simulink model "LTI_vs_LPV_vs_NL_realimentado_NL"  (R2020a)
settings: Solver=VariableStepAuto  StartTime=0.0  StopTime=10.0  RelTol=1e-3
values from neighbouring files (symbols this model uses):
  A = [ 0        1               0 ... (first row only)    [AnalisisDeEstabilidad.m]    (also in Consigna_de_pos.m = [t_1^3,t_1^2,t_1,1; Controlabilidad.m = [0 ,       1      ,         0; Funciones_de_Transferencia.m = [ 0         1                           0; LTI_vs_LPV_vs_NL_realimentado.m = [0                                                       1  )
  alpha_cu = 3.9e-3    (= 0.0039)    [AnalisisDeEstabilidad.m]    (also in LTI_vs_LPV_vs_NL_realimentado.m; Modelo_linealizado.m)
  B = [0              0 ... (first row only)    [AnalisisDeEstabilidad.m]    (also in Consigna_de_pos.m = [theta_m1; theta_m2; 0 ;0]; Controlabilidad.m = [0;0;1/Lq]; LTI_vs_LPV_vs_NL_realimentado.m = [0      0       0           0           0; Modelo_linealizado.m = [0,0,0,0,0)
  b_eq = b_m + b_l/(r^2)    (= 2.19444444444e-05)    [LTI_vs_LPV_vs_NL_realimentado.m]    (also in Modelo_linealizado.m)
  C_ts = 0.818    [LTI_vs_LPV_vs_NL_realimentado.m]    (also in Modelo_linealizado.m)
  i_0s_o = double(solutions.i_0so(1))    [LTI_vs_LPV_vs_NL_realimentado.m]
  i_ds_o = double(solutions.i_tot(1)*cos(beta))    [LTI_vs_LPV_vs_NL_realimentado.m]    (also in Modelo_linealizado.m = 0)
  i_qs_o = double(solutions.i_tot(1)*sin(beta))    [LTI_vs_LPV_vs_NL_realimentado.m]    (also in Modelo_linealizado.m = 0)
  J_eq = J_m + J_l/(r^2)    (= 1.97847222222e-05)    [LTI_vs_LPV_vs_NL_realimentado.m]    (also in Modelo_linealizado.m)
  L_d = 6.6/1000    (= 0.0066)    [Curvas_carc.m]    (also in LTI_vs_LPV_vs_NL_realimentado.m; Modelo_linealizado.m)
  L_ls = 0.8/1000    (= 0.0008)    [LTI_vs_LPV_vs_NL_realimentado.m]    (also in Modelo_linealizado.m)
  L_q = 5.8/1000    (= 0.0058)    [Curvas_carc.m]    (also in LTI_vs_LPV_vs_NL_realimentado.m; Modelo_linealizado.m)
  lambda_m = 0.01546    [Curvas_carc.m]    (also in LTI_vs_LPV_vs_NL_realimentado.m = 0.016; Modelo_linealizado.m = 0.016)
  omega_m_o = double(solutions.omega_mo(1))    [LTI_vs_LPV_vs_NL_realimentado.m]    (also in Modelo_linealizado.m = 0)
  P_p = 3    [Curvas_carc.m]    (also in LTI_vs_LPV_vs_NL_realimentado.m)
  Pp = 3    [AnalisisDeEstabilidad.m]    (also in LTI_vs_LPV_vs_NL_realimentado.m; Modelo_linealizado.m; parametros.m)
  r = 120    [AnalisisDeEstabilidad.m]    (also in LTI_vs_LPV_vs_NL_realimentado.m; Modelo_linealizado.m; parametros.m)
  R_s = 1.02    [Curvas_carc.m]    (also in LTI_vs_LPV_vs_NL_realimentado.m = R_s_o; Modelo_linealizado.m = 0.348)
  R_sREF = R_sref    (= 1.02)    [LTI_vs_LPV_vs_NL_realimentado.m]
  R_ts_amb = 146.7    [LTI_vs_LPV_vs_NL_realimentado.m]    (also in Modelo_linealizado.m)
  T_amb = T_amb_o    (= 25)    [LTI_vs_LPV_vs_NL_realimentado.m]
  T_amb_o = 25    [LTI_vs_LPV_vs_NL_realimentado.m]    (also in Modelo_linealizado.m = -15:10:40)
  T_l_o = 0    [LTI_vs_LPV_vs_NL_realimentado.m]
  T_s_o = double(solutions.T_so(1))    [LTI_vs_LPV_vs_NL_realimentado.m]    (also in Modelo_linealizado.m = 40)
  T_sREF = T_sref    (= 40)    [LTI_vs_LPV_vs_NL_realimentado.m]
  theta_m_o = r*pi/12    (= 31.4159265359)    [LTI_vs_LPV_vs_NL_realimentado.m]    (also in Modelo_linealizado.m = 0)
  v_0s = v_0s_o    (= 0)    [LTI_vs_LPV_vs_NL_realimentado.m]    (also in Modelo_linealizado.m)
  v_0s_o = 0    [LTI_vs_LPV_vs_NL_realimentado.m]
  v_ds = 10    [Curvas_carc.m]    (also in LTI_vs_LPV_vs_NL_realimentado.m = 0)
  v_ds_o = double(solutions.v_dso(1))    [LTI_vs_LPV_vs_NL_realimentado.m]
  v_qs_o = double(solutions.v_qso(1))    [LTI_vs_LPV_vs_NL_realimentado.m]
undefined symbols (not defined in the file or in its folder): sigbuilder_block
settings Model: Creator=Juan  LastModifiedBy=Juan

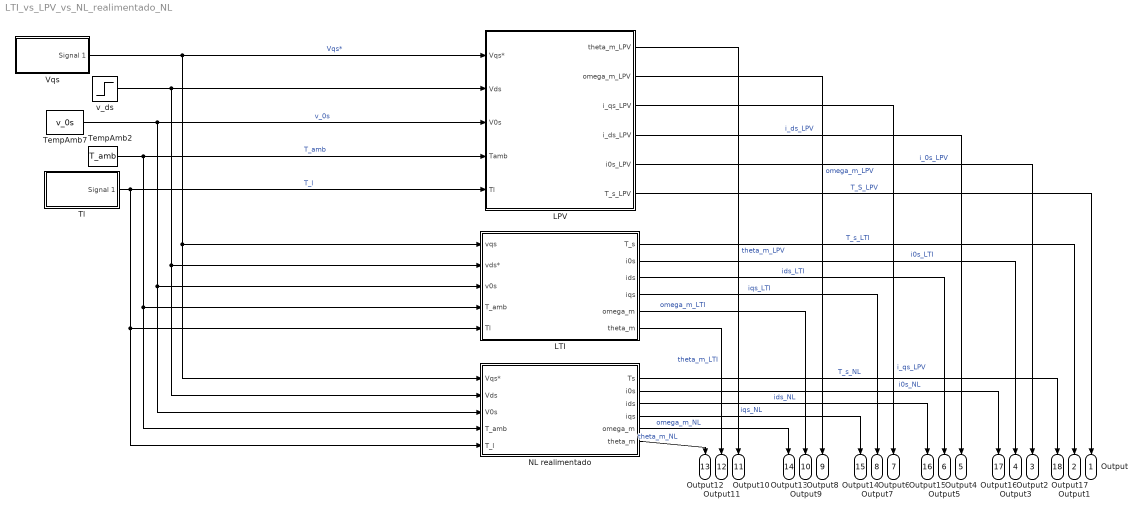
== system LTI_vs_LPV_vs_NL_realimentado_NL ==
  LPV : Subsystem
  LTI : Subsystem
  NL realimentado : Subsystem
  TempAmb2 : Constant  Value=T_amb
  TempAmb7 : Constant  Value=v_0s
  Tl : Subsystem  Tag=STV Subsys  LoadFcn=sigbuilder_block('load');  StartFcn=sigbuilder_block('start');  StopFcn=sigbuilder_block('stop');  ClipboardFcn=sigbuilder_block('clipboard');  mask(Sigbuilder block){tuvar=[0:10]}
      mask help: Simulink:masks:SigbuilderBlock_MD
      mask init:
      | if ~strcmp(get_param(bdroot(gcbh),'SimulationStatus'),'stopped') tuvar = sigbuilder_block('maskInit'); end
      settings: CopyFcn=sigbuilder_block('copy');  DeleteFcn=sigbuilder_block('delete');  ModelCloseFcn=sigbuilder_block('modelClose');  PreSaveFcn=sigbuilder_block('preSave');  PauseFcn=sigbuilder_block('pause');  ContinueFcn=sigbuilder_block('continue');  NameChangeFcn=sigbuilder_block('namechange');  OpenFcn=sigbuilder_block('open',[0 36 1152 555.6 ]);  CloseFcn=sigbuilder_block('close');
      mask Display: plot(0, 0, 100, 100,[2, 2, 32, 32, 2], [68, 8, 8, 68, 68],[32, 2], [38, 38], [32, 19, 2],[53, 60, 44], [32, 17, 17, 2],[16, 16, 31, 31]);txt = getActiveGroup(gcbh);text(2, 100, txt,'verticalAlignment', 'top');
  Vqs : Subsystem  Tag=STV Subsys  LoadFcn=sigbuilder_block('load');  StartFcn=sigbuilder_block('start');  StopFcn=sigbuilder_block('stop');  ClipboardFcn=sigbuilder_block('clipboard');  mask(Sigbuilder block){tuvar=[0:10]}
      mask help: Simulink:masks:SigbuilderBlock_MD
      mask init:
      | if ~strcmp(get_param(bdroot(gcbh),'SimulationStatus'),'stopped') tuvar = sigbuilder_block('maskInit'); end
      settings: CopyFcn=sigbuilder_block('copy');  DeleteFcn=sigbuilder_block('delete');  ModelCloseFcn=sigbuilder_block('modelClose');  PreSaveFcn=sigbuilder_block('preSave');  PauseFcn=sigbuilder_block('pause');  ContinueFcn=sigbuilder_block('continue');  NameChangeFcn=sigbuilder_block('namechange');  OpenFcn=sigbuilder_block('open',[5.4 36 1141.2 516.6 ]);  CloseFcn=sigbuilder_block('close');
      mask Display: plot(0, 0, 100, 100,[2, 2, 32, 32, 2], [68, 8, 8, 68, 68],[32, 2], [38, 38], [32, 19, 2],[53, 60, 44], [32, 17, 17, 2],[16, 16, 31, 31]);txt = getActiveGroup(gcbh);text(2, 100, txt,'verticalAlignment', 'top');
  v_ds : Step  After=v_ds  SampleTime=0
  Output : Outport
  Output1 : Outport  Port=2
  Output2 : Outport  Port=3
  Output3 : Outport  Port=4
  Output4 : Outport  Port=5
  Output5 : Outport  Port=6
  Output6 : Outport  Port=7
  Output7 : Outport  Port=8
  Output8 : Outport  Port=9
  Output9 : Outport  Port=10
  Output10 : Outport  Port=11
  Output11 : Outport  Port=12
  Output12 : Outport  Port=13
  Output13 : Outport  Port=14
  Output14 : Outport  Port=15
  Output15 : Outport  Port=16
  Output16 : Outport  Port=17
  Output17 : Outport  Port=18
  wires:
  LTI/3(ids) -> Output5/1  "ids_LTI"
  LTI/5(omega_m) -> Output9/1  "omega_m_LTI"
  LTI/1(T_s) -> Output1/1  "T_s_LTI"
  LTI/4(iqs) -> Output7/1  "iqs_LTI"
  LTI/2(i0s) -> Output3/1  "i0s_LTI"
  TempAmb7/1 -> NL realimentado/3(V0s), LTI/3(v0s), LPV/3(V0s)  "v_0s"
  TempAmb2/1 -> NL realimentado/4(T_amb), LTI/4(T_amb), LPV/4(Tamb)  "T_amb"
  LTI/6(theta_m) -> Output11/1  "theta_m_LTI"
  v_ds/1 -> NL realimentado/2(Vds), LTI/2(vds*), LPV/2(Vds)
  Tl/1(Signal 1) -> LPV/5(Tl), NL realimentado/5(T_l), LTI/5(Tl)  "T_l"
  Vqs/1(Signal 1) -> NL realimentado/1(Vqs*), LTI/1(vqs), LPV/1(Vqs*)  "Vqs*"
  LPV/1(theta_m_LPV) -> Output10/1  "theta_m_LPV"
  LPV/2(omega_m_LPV) -> Output8/1  "omega_m_LPV"
  LPV/3(i_qs_LPV) -> Output6/1  "i_qs_LPV"
  LPV/4(i_ds_LPV) -> Output4/1  "i_ds_LPV"
  LPV/5(i0s_LPV) -> Output2/1  "i_0s_LPV"
  LPV/6(T_s_LPV) -> Output/1  "T_S_LPV"
  NL realimentado/6(theta_m) -> Output12/1  "theta_m_NL"
  NL realimentado/5(omega_m) -> Output13/1  "omega_m_NL"
  NL realimentado/4(iqs) -> Output14/1  "iqs_NL"
  NL realimentado/3(ids) -> Output15/1  "ids_NL"
  NL realimentado/2(i0s) -> Output16/1  "i0s_NL"
  NL realimentado/1(Ts) -> Output17/1  "T_s_NL"

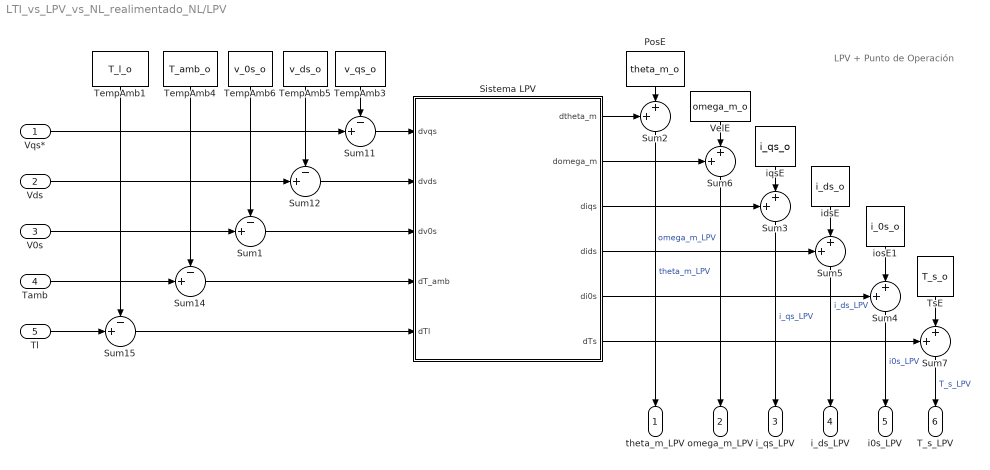
== system LTI_vs_LPV_vs_NL_realimentado_NL/LPV ==
  note: LPV + Punto de Operación
  Vqs* : Inport
  Vds : Inport  Port=2
  V0s : Inport  Port=3
  Tamb : Inport  Port=4
  Tl : Inport  Port=5
  PosE : Constant  Value=theta_m_o
  Sistema LPV : Subsystem
  Sum{1,11..12,14..15} (5 alike) : Sum  Inputs=-+|
  Sum{2..7} (6 alike) : Sum  Inputs=++|
  TempAmb1 : Constant  Value=T_l_o
  TempAmb3 : Constant  Value=v_qs_o
  TempAmb4 : Constant  Value=T_amb_o
  TempAmb5 : Constant  Value=v_ds_o
  TempAmb6 : Constant  Value=v_0s_o
  TsE : Constant  Value=T_s_o
  VelE : Constant  Value=omega_m_o
  idsE : Constant  Value=i_ds_o
  iosE1 : Constant  Value=i_0s_o
  iqsE : Constant  Value=i_qs_o
  theta_m_LPV : Outport
  omega_m_LPV : Outport  Port=2
  i_qs_LPV : Outport  Port=3
  i_ds_LPV : Outport  Port=4
  i0s_LPV : Outport  Port=5
  T_s_LPV : Outport  Port=6
  wires:
  V0s/1 -> Sum1/2
  Sum12/1 -> Sistema LPV/2(dvds)
  Sum1/1 -> Sistema LPV/3(dv0s)
  Sum5/1 -> i_ds_LPV/1  "i_ds_LPV"
  iosE1/1 -> Sum4/2
  TempAmb4/1 -> Sum14/1
  Sistema LPV/4(dids) -> Sum5/1
  TempAmb6/1 -> Sum1/1
  Tamb/1 -> Sum14/2
  iqsE/1 -> Sum3/2
  TsE/1 -> Sum7/2
  TempAmb5/1 -> Sum12/1
  idsE/1 -> Sum5/2
  TempAmb1/1 -> Sum15/1
  Sum14/1 -> Sistema LPV/4(dT_amb)
  Sistema LPV/6(dTs) -> Sum7/1
  Sum11/1 -> Sistema LPV/1(dvqs)
  Sistema LPV/2(domega_m) -> Sum6/1
  Sum15/1 -> Sistema LPV/5(dTl)
  Sistema LPV/5(di0s) -> Sum4/1
  Vds/1 -> Sum12/2
  VelE/1 -> Sum6/2
  Sum6/1 -> omega_m_LPV/1  "omega_m_LPV"
  PosE/1 -> Sum2/2
  Sistema LPV/1(dtheta_m) -> Sum2/1
  Sistema LPV/3(diqs) -> Sum3/1
  TempAmb3/1 -> Sum11/1
  Tl/1 -> Sum15/2
  Sum4/1 -> i0s_LPV/1  "i0s_LPV"
  Sum3/1 -> i_qs_LPV/1  "i_qs_LPV"
  Sum2/1 -> theta_m_LPV/1  "theta_m_LPV"
  Sum7/1 -> T_s_LPV/1  "T_s_LPV"
  Vqs*/1 -> Sum11/2

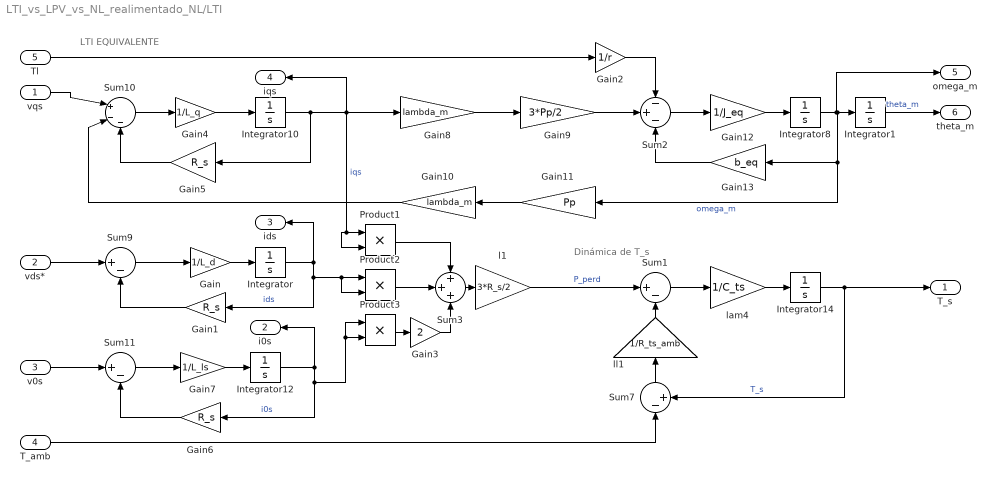
== system LTI_vs_LPV_vs_NL_realimentado_NL/LTI ==
  note: Dinámica de T_s
  note: LTI EQUIVALENTE
  vqs : Inport
  vds* : Inport  Port=2
  v0s : Inport  Port=3
  T_amb : Inport  Port=4
  Tl : Inport  Port=5
  Gain : Gain  Gain=1/L_d
  Gain1 : Gain  Gain=R_s
  Gain10 : Gain  Gain=lambda_m
  Gain11 : Gain  Gain=Pp
  Gain12 : Gain  Gain=1/J_eq
  Gain13 : Gain  Gain=b_eq
  Gain2 : Gain  Gain=1/r
  Gain3 : Gain  Gain=2
  Gain4 : Gain  Gain=1/L_q
  Gain5 : Gain  Gain=R_s
  Gain6 : Gain  Gain=R_s
  Gain7 : Gain  Gain=1/L_ls
  Gain8 : Gain  Gain=lambda_m
  Gain9 : Gain  Gain=3*Pp/2
  Integrator{,1,8,10,12} (5 alike) : Integrator
  Integrator14 : Integrator  InitialCondition=T_amb
  Product1 : Product
  Product2 : Product
  Product3 : Product
  Sum1 : Sum  Inputs=|+-
  Sum10 : Sum  Inputs=|+--
  Sum11 : Sum  Inputs=|+-
  Sum2 : Sum  Inputs=-+-
  Sum3 : Sum  Inputs=+++
  Sum7 : Sum  Inputs=|-+
  Sum9 : Sum  Inputs=|+-
  l1 : Gain  Gain=3*R_s/2
  lam4 : Gain  Gain=1/C_ts
  ll1 : Gain  Gain=1/R_ts_amb
  T_s : Outport
  i0s : Outport  Port=2
  ids : Outport  Port=3
  iqs : Outport  Port=4
  omega_m : Outport  Port=5
  theta_m : Outport  Port=6
  wires:
  Integrator/1 -> ids/1, Gain1/1, Product2/2, Product2/1  "ids"
  Sum7/1 -> ll1/1
  Gain5/1 -> Sum10/3
  Sum11/1 -> Gain7/1
  Gain7/1 -> Integrator12/1
  Product1/1 -> Sum3/1
  Gain13/1 -> Sum2/3
  Integrator8/1 -> omega_m/1, Integrator1/1, Gain11/1, Gain13/1  "omega_m"
  Gain6/1 -> Sum11/2
  Gain4/1 -> Integrator10/1
  Gain8/1 -> Gain9/1
  Gain/1 -> Integrator/1
  Integrator12/1 -> Product3/1, Product3/2, Gain6/1, i0s/1  "i0s"
  Integrator10/1 -> Product1/2, Product1/1, iqs/1, Gain8/1, Gain5/1  "iqs"
  Gain1/1 -> Sum9/2
  Tl/1 -> Gain2/1
  v0s/1 -> Sum11/1
  Gain11/1 -> Gain10/1
  lam4/1 -> Integrator14/1
  Gain10/1 -> Sum10/2
  T_amb/1 -> Sum7/1
  Gain2/1 -> Sum2/1
  Sum1/1 -> lam4/1
  Integrator14/1 -> Sum7/2, T_s/1  "T_s"
  l1/1 -> Sum1/1  "P_perd"
  vds*/1 -> Sum9/1
  Gain12/1 -> Integrator8/1
  Product2/1 -> Sum3/2
  Sum9/1 -> Gain/1
  Gain3/1 -> Sum3/3
  Gain9/1 -> Sum2/2
  Integrator1/1 -> theta_m/1  "theta_m"
  Product3/1 -> Gain3/1
  vqs/1 -> Sum10/1
  Sum2/1 -> Gain12/1
  Sum10/1 -> Gain4/1
  ll1/1 -> Sum1/2
  Sum3/1 -> l1/1

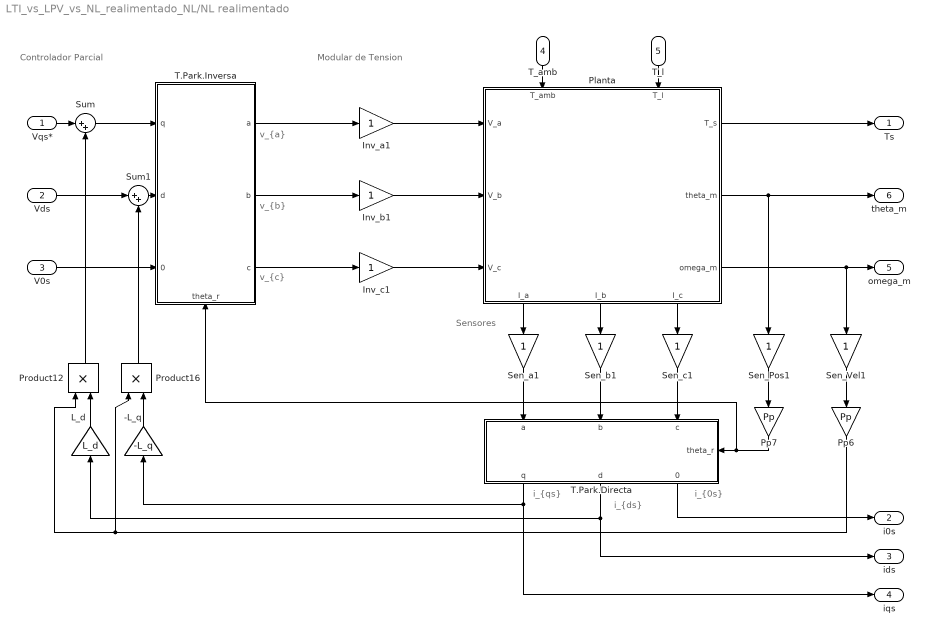
== system LTI_vs_LPV_vs_NL_realimentado_NL/NL realimentado ==
  note: i_{qs}
  note: i_{ds}
  note: Modular de Tension
  note: v_{c}
  note: Controlador Parcial
  note: Sensores
  note: v_{a}
  note: i_{0s}
  note: v_{b}
  Vqs* : Inport
  Vds : Inport  Port=2
  V0s : Inport  Port=3
  T_amb : Inport  Port=4
  T_l : Inport  Port=5
  -L_q : Gain  Gain=-L_q
  Inv_a1 : Gain
  Inv_b1 : Gain
  Inv_c1 : Gain
  L_d : Gain  Gain=L_d
  Planta : Subsystem
      settings: PortSchema="{\"entries\":[{\"content\":{\"sides\":[{\"content\":{\"connectorIds\":[\"In1\",\"In2\",\"In3\"]},\"type\":\"ConnectorPlacement.EquallySpacedRectSide\",\"uuid\":\"baf32630-7abf-43de-8d1d-ef19bce8ef09\"},{\"content\":{\"connectorIds\":[\"Out1\",\"Out2\",\"Out3\"],\"side\":\"RIGHT\"},\"type\":\"ConnectorPlacement.EquallySpacedRectSide\",\"uuid\":\"8343cc29-d6ed-46ed-8bbc-86cce19f52c3\"},{\"content\":{\"connectorIds\":[\"In4\",\"In5\"],\"side\":\"TOP\"},\"type\":\"ConnectorPlacement.EquallySpacedRectSide\",\"uuid\":\"0b8be76f-f25b-4801-8835-92ed2105f393\"},{\"content\":{\"connectorIds\":[\"Out4\",\"Out5\",\"Out6\"],\"side\":\"BOTTOM\"},\"type\":\"ConnectorPlacement.EquallySpacedRectSide\",\"uuid\":\"fe3e13b1-008f-430e-9d12-27931368b9b5\"}]},\"type\":\"ConnectorPlacement.EquallySpacedConnector\",\"uuid\":\"84d47617-2d56-43e0-a9a1-133a35a1552a\"}],\"packageUris\":[\"http://schema.mathworks.com/mf0/Connector/19700101\"],\"version\":\"1.0\"}"
  Pp6 : Gain  Gain=Pp
  Pp7 : Gain  Gain=Pp
  Product12 : Product
  Product16 : Product
  Sen_Pos1 : Gain
  Sen_Vel1 : Gain
  Sen_a1 : Gain
  Sen_b1 : Gain
  Sen_c1 : Gain
  Sum : Sum  Inputs=|++
  Sum1 : Sum  Inputs=|++
  T.Park.Directa : Subsystem
      settings: PortSchema="{\"entries\":[{\"content\":{\"sides\":[{\"content\":{\"connectorIds\":[\"In1\",\"In2\",\"In3\"]},\"type\":\"ConnectorPlacement.EquallySpacedRectSide\",\"uuid\":\"2bfbe7ef-652a-4797-b13c-b84c243bd68c\"},{\"content\":{\"connectorIds\":[\"Out1\",\"Out2\",\"Out3\"],\"side\":\"RIGHT\"},\"type\":\"ConnectorPlacement.EquallySpacedRectSide\",\"uuid\":\"075def0e-c436-44dc-ba25-82cf6ffae869\"},{\"content\":{\"connectorIds\":[],\"side\":\"TOP\"},\"type\":\"ConnectorPlacement.EquallySpacedRectSide\",\"uuid\":\"95d81334-e332-4f04-a2cb-c4692f91809c\"},{\"content\":{\"connectorIds\":[\"In4\"],\"side\":\"BOTTOM\"},\"type\":\"ConnectorPlacement.EquallySpacedRectSide\",\"uuid\":\"85b95360-e43d-49d1-a18f-690334b045e6\"}]},\"type\":\"ConnectorPlacement.EquallySpacedConnector\",\"uuid\":\"b90f9cad-0277-459c-bcac-17172872a787\"}],\"packageUris\":[\"http://schema.mathworks.com/mf0/Connector/19700101\"],\"version\":\"1.0\"}"
  T.Park.Inversa : Subsystem
      settings: PortSchema="{\"entries\":[{\"content\":{\"sides\":[{\"content\":{\"connectorIds\":[\"In1\",\"In2\",\"In3\"]},\"type\":\"ConnectorPlacement.EquallySpacedRectSide\",\"uuid\":\"a662f436-bc73-44f7-82e0-06261d9ef40c\"},{\"content\":{\"connectorIds\":[\"Out1\",\"Out2\",\"Out3\"],\"side\":\"RIGHT\"},\"type\":\"ConnectorPlacement.EquallySpacedRectSide\",\"uuid\":\"409fe548-c31d-4794-9ee2-a38875bf0027\"},{\"content\":{\"connectorIds\":[],\"side\":\"TOP\"},\"type\":\"ConnectorPlacement.EquallySpacedRectSide\",\"uuid\":\"438665e9-fbd8-4951-83da-f4b2ee30dc53\"},{\"content\":{\"connectorIds\":[\"In4\"],\"side\":\"BOTTOM\"},\"type\":\"ConnectorPlacement.EquallySpacedRectSide\",\"uuid\":\"8fba0a52-96af-41e4-9875-ca52b7a9f572\"}]},\"type\":\"ConnectorPlacement.EquallySpacedConnector\",\"uuid\":\"9855907b-9604-47a6-98ae-3aa5d30a95f1\"}],\"packageUris\":[\"http://schema.mathworks.com/mf0/Connector/19700101\"],\"version\":\"1.0\"}"
  Ts : Outport
  i0s : Outport  Port=2
  ids : Outport  Port=3
  iqs : Outport  Port=4
  omega_m : Outport  Port=5
  theta_m : Outport  Port=6
  wires:
  Inv_c1/1 -> Planta/3(V_c)
  Planta/2(theta_m) -> theta_m/1, Sen_Pos1/1
  -L_q/1 -> Product16/2
  T.Park.Directa/1(q) -> iqs/1, -L_q/1
  Planta/6(I_c) -> Sen_c1/1
  Planta/3(omega_m) -> Sen_Vel1/1, omega_m/1
  V0s/1 -> T.Park.Inversa/3(0)
  Sen_Vel1/1 -> Pp6/1
  Vqs*/1 -> Sum/1
  Product12/1 -> Sum/2
  Sen_c1/1 -> T.Park.Directa/3(c)
  T.Park.Inversa/1(a) -> Inv_a1/1
  Planta/1(T_s) -> Ts/1
  T.Park.Inversa/2(b) -> Inv_b1/1
  Sen_Pos1/1 -> Pp7/1
  Inv_b1/1 -> Planta/2(V_b)
  T_amb/1 -> Planta/4(T_amb)
  T.Park.Inversa/3(c) -> Inv_c1/1
  Planta/4(I_a) -> Sen_a1/1
  Sen_a1/1 -> T.Park.Directa/1(a)
  Planta/5(I_b) -> Sen_b1/1
  Pp7/1 -> T.Park.Inversa/4(theta_r), T.Park.Directa/4(theta_r)
  Inv_a1/1 -> Planta/1(V_a)
  L_d/1 -> Product12/2
  T.Park.Directa/2(d) -> ids/1, L_d/1
  Sum/1 -> T.Park.Inversa/1(q)
  Pp6/1 -> Product16/1, Product12/1
  Sen_b1/1 -> T.Park.Directa/2(b)
  T.Park.Directa/3(0) -> i0s/1
  Product16/1 -> Sum1/2
  Sum1/1 -> T.Park.Inversa/2(d)
  Vds/1 -> Sum1/1
  T_l/1 -> Planta/5(T_l)

== system LTI_vs_LPV_vs_NL_realimentado_NL/Tl ==
  Demux : Demux  Tag=STV Demux  Outputs=1
      settings: DisplayOption=none
  FromWs : FromWorkspace  Tag=STV FromWs  VariableName=tuvar
      SigBuilderData=|
      | common.afterFinalStr = 'Extrapolate'
      | common.sampleTime = 0
      | dataSet.timeRange = [0 10]
      | dataSet.name = 'Group 1'
      | sbobj.Groups.Name = 'Group 1'
      | sbobj.Groups.Signals.Name = 'Signal 1'
      | sbobj.Groups.Signals.XData = [0 0.3 0.3 0.5 0.5 0.9 0.9 10]
      | sbobj.Groups.Signals.YData = [0 0 6.28 6.28 -6.28 -6.28 0 0]
  Signal 1 : Outport  Tag=STV Outport
  wires:
  Demux/1 -> Signal 1/1
  FromWs/1 -> Demux/1

== system LTI_vs_LPV_vs_NL_realimentado_NL/Vqs ==
  Demux : Demux  Tag=STV Demux  Outputs=1
      settings: DisplayOption=none
  FromWs : FromWorkspace  Tag=STV FromWs  VariableName=tuvar
      SigBuilderData=|
      | common.afterFinalStr = 'Extrapolate'
      | common.sampleTime = 0
      | dataSet.timeRange = [0 10]
      | dataSet.name = 'Group 1'
      | sbobj.Groups.Name = 'Group 1'
      | sbobj.Groups.Signals.Name = 'Signal 1'
      | sbobj.Groups.Signals.XData = [0 0.1 0.1 0.7 0.7 10]
      | sbobj.Groups.Signals.YData = [0 0 19.596 19.596 0 0]
  Signal 1 : Outport  Tag=STV Outport
  wires:
  Demux/1 -> Signal 1/1
  FromWs/1 -> Demux/1

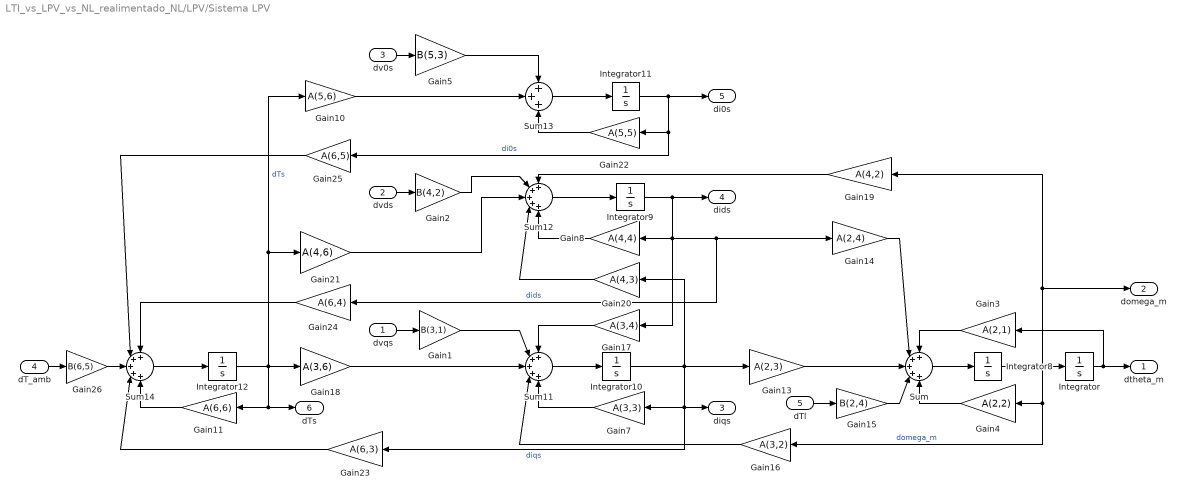
== system LTI_vs_LPV_vs_NL_realimentado_NL/LPV/Sistema LPV ==
  dvqs : Inport
  dvds : Inport  Port=2
  dv0s : Inport  Port=3
  dT_amb : Inport  Port=4
  dTl : Inport  Port=5
  Gain1 : Gain  Gain=B(3,1)
  Gain10 : Gain  Gain=A(5,6)
  Gain11 : Gain  Gain=A(6,6)
  Gain13 : Gain  Gain=A(2,3)
  Gain14 : Gain  Gain=A(2,4)
  Gain15 : Gain  Gain=B(2,4)
  Gain16 : Gain  Gain=A(3,2)
  Gain17 : Gain  Gain=A(3,4)
  Gain18 : Gain  Gain=A(3,6)
  Gain19 : Gain  Gain=A(4,2)
  Gain2 : Gain  Gain=B(4,2)
  Gain20 : Gain  Gain=A(4,3)
  Gain21 : Gain  Gain=A(4,6)
  Gain22 : Gain  Gain=A(5,5)
  Gain23 : Gain  Gain=A(6,3)
  Gain24 : Gain  Gain=A(6,4)
  Gain25 : Gain  Gain=A(6,5)
  Gain26 : Gain  Gain=B(6,5)
  Gain3 : Gain  Gain=A(2,1)
  Gain4 : Gain  Gain=A(2,2)
  Gain5 : Gain  Gain=B(5,3)
  Gain7 : Gain  Gain=A(3,3)
  Gain8 : Gain  Gain=A(4,4)
  Integrator{,8..12} (6 alike) : Integrator
  Sum{,11..12,14} (4 alike) : Sum  Inputs=+++++
  Sum13 : Sum  Inputs=+++
  dtheta_m : Outport
  domega_m : Outport  Port=2
  diqs : Outport  Port=3
  dids : Outport  Port=4
  di0s : Outport  Port=5
  dTs : Outport  Port=6
  wires:
  dTl/1 -> Gain15/1
  Integrator/1 -> dtheta_m/1, Gain3/1
  Integrator9/1 -> dids/1, Gain8/1, Gain17/1, Gain24/1, Gain14/1  "dids"
  Integrator10/1 -> Gain20/1, Gain13/1, Gain23/1, Gain7/1, diqs/1  "diqs"
  Gain25/1 -> Sum14/2
  Integrator11/1 -> di0s/1, Gain25/1, Gain22/1  "di0s"
  Sum13/1 -> Integrator11/1
  Gain13/1 -> Sum/3
  Gain24/1 -> Sum14/1
  Integrator8/1 -> Gain16/1, Gain4/1, Gain19/1, domega_m/1, Integrator/1  "domega_m"
  Sum12/1 -> Integrator9/1
  Integrator12/1 -> dTs/1, Gain11/1, Gain18/1, Gain10/1, Gain21/1  "dTs"
  Gain15/1 -> Sum/4
  Gain18/1 -> Sum11/3
  Sum11/1 -> Integrator10/1
  Gain20/1 -> Sum12/4
  dT_amb/1 -> Gain26/1
  Gain14/1 -> Sum/2
  Sum14/1 -> Integrator12/1
  Gain8/1 -> Sum12/5
  Gain26/1 -> Sum14/3
  Gain23/1 -> Sum14/4
  Gain21/1 -> Sum12/3
  Gain16/1 -> Sum11/4
  dv0s/1 -> Gain5/1
  Gain19/1 -> Sum12/1
  Sum/1 -> Integrator8/1
  Gain17/1 -> Sum11/1
  dvqs/1 -> Gain1/1
  Gain22/1 -> Sum13/3
  Gain11/1 -> Sum14/5
  dvds/1 -> Gain2/1
  Gain10/1 -> Sum13/2
  Gain1/1 -> Sum11/2
  Gain2/1 -> Sum12/2
  Gain3/1 -> Sum/1
  Gain4/1 -> Sum/5
  Gain7/1 -> Sum11/5
  Gain5/1 -> Sum13/1

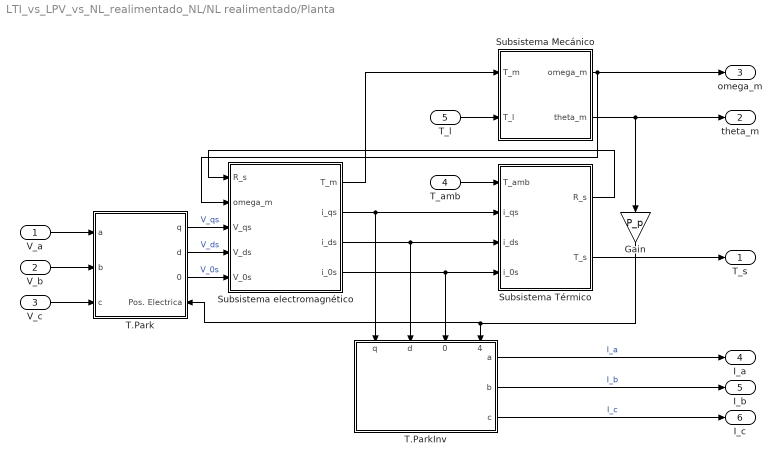
== system LTI_vs_LPV_vs_NL_realimentado_NL/NL realimentado/Planta ==
  V_a : Inport
  V_b : Inport  Port=2
  V_c : Inport  Port=3
  T_amb : Inport  Port=4
  T_l : Inport  Port=5
  "\tSubsistema Térmico" : Subsystem
  Gain : Gain  Gain=P_p
  Subsistema Mecánico : Subsystem
  Subsistema electromagnético : Subsystem
  T.Park : Subsystem
      settings: PortSchema="{\"entries\":[{\"content\":{\"sides\":[{\"content\":{\"connectorIds\":[\"In1\",\"In2\",\"In3\"]},\"type\":\"ConnectorPlacement.EquallySpacedRectSide\",\"uuid\":\"2bfbe7ef-652a-4797-b13c-b84c243bd68c\"},{\"content\":{\"connectorIds\":[\"Out1\",\"Out2\",\"Out3\",\"In4\"],\"side\":\"RIGHT\"},\"type\":\"ConnectorPlacement.EquallySpacedRectSide\",\"uuid\":\"075def0e-c436-44dc-ba25-82cf6ffae869\"},{\"content\":{\"connectorIds\":[],\"side\":\"TOP\"},\"type\":\"ConnectorPlacement.EquallySpacedRectSide\",\"uuid\":\"95d81334-e332-4f04-a2cb-c4692f91809c\"}]},\"type\":\"ConnectorPlacement.EquallySpacedConnector\",\"uuid\":\"b90f9cad-0277-459c-bcac-17172872a787\"}],\"packageUris\":[\"http://schema.mathworks.com/mf0/Connector/19700101\"],\"version\":\"1.0\"}"
  T.ParkInv : Subsystem
      settings: PortSchema="{\"entries\":[{\"content\":{\"sides\":[{\"content\":{\"connectorIds\":[\"In1\",\"In2\",\"In3\",\"In4\"]},\"type\":\"ConnectorPlacement.EquallySpacedRectSide\",\"uuid\":\"aef3590a-5fc0-4a95-8f41-1fc79c0f3fe7\"},{\"content\":{\"connectorIds\":[],\"side\":\"RIGHT\"},\"type\":\"ConnectorPlacement.EquallySpacedRectSide\",\"uuid\":\"4e7c387b-9bca-48cc-a151-2357bd6b7b1d\"},{\"content\":{\"connectorIds\":[],\"side\":\"TOP\"},\"type\":\"ConnectorPlacement.EquallySpacedRectSide\",\"uuid\":\"1231932f-f9d3-49e6-b404-2af91cb220c6\"},{\"content\":{\"connectorIds\":[\"Out1\",\"Out2\",\"Out3\"],\"side\":\"BOTTOM\"},\"type\":\"ConnectorPlacement.EquallySpacedRectSide\",\"uuid\":\"4f29e626-7677-496e-bb82-59a3ecbc7a95\"}]},\"type\":\"ConnectorPlacement.EquallySpacedConnector\",\"uuid\":\"48e39a78-817d-4753-b518-4d689d2c1635\"}],\"packageUris\":[\"http://schema.mathworks.com/mf0/Connector/19700101\"],\"version\":\"1.0\"}"
  T_s : Outport
  theta_m : Outport  Port=2
  omega_m : Outport  Port=3
  I_a : Outport  Port=4
  I_b : Outport  Port=5
  I_c : Outport  Port=6
  wires:
  Subsistema Mecánico/2(theta_m) -> Gain/1, theta_m/1
  Gain/1 -> T.Park/4(Pos. Electrica), T.ParkInv/4(Pos. Electrica)
  T.Park/1(q) -> Subsistema electromagnético/3(V_qs)  "V_qs"
  Subsistema Mecánico/1(omega_m) -> Subsistema electromagnético/2(omega_m), omega_m/1
  Subsistema electromagnético/2(i_qs) -> "\tSubsistema Térmico"/2(i_qs), T.ParkInv/1(q)
  Subsistema electromagnético/1(T_m) -> Subsistema Mecánico/1(T_m)
  Subsistema electromagnético/4(i_0s) -> "\tSubsistema Térmico"/4(i_0s), T.ParkInv/3(0)
  V_c/1 -> T.Park/3(c)
  T.ParkInv/3(c) -> I_c/1  "I_c"
  T.ParkInv/2(b) -> I_b/1  "I_b"
  Subsistema electromagnético/3(i_ds) -> "\tSubsistema Térmico"/3(i_ds), T.ParkInv/2(d)
  V_b/1 -> T.Park/2(b)
  T.ParkInv/1(a) -> I_a/1  "I_a"
  T.Park/3(0) -> Subsistema electromagnético/5(V_0s)  "V_0s"
  V_a/1 -> T.Park/1(a)
  T.Park/2(d) -> Subsistema electromagnético/4(V_ds)  "V_ds"
  T_l/1 -> Subsistema Mecánico/2(T_l)
  T_amb/1 -> "\tSubsistema Térmico"/1(T_amb)
  "\tSubsistema Térmico"/1(R_s) -> Subsistema electromagnético/1(R_s)
  "\tSubsistema Térmico"/2(T_s) -> T_s/1

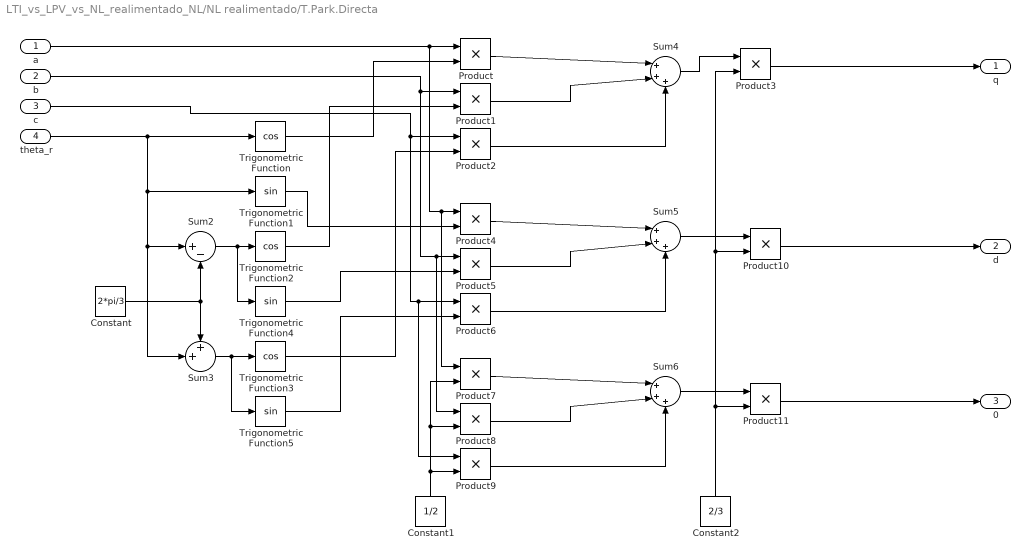
== system LTI_vs_LPV_vs_NL_realimentado_NL/NL realimentado/T.Park.Directa ==
  a : Inport
  b : Inport  Port=2
  c : Inport  Port=3
  theta_r : Inport  Port=4
  Constant : Constant  Value=2*pi/3
  Constant1 : Constant  Value=1/2
  Constant2 : Constant  Value=2/3
  Product{,1..11} (12 alike) : Product
  Sum2 : Sum  Inputs=|+-
  Sum3 : Sum  Inputs=++|
  Sum4 : Sum  Inputs=|+++
  Sum5 : Sum  Inputs=|+++
  Sum6 : Sum  Inputs=|+++
  Trigonometric Function : Trigonometry  Operator=cos
  Trigonometric Function1 : Trigonometry
  Trigonometric Function2 : Trigonometry  Operator=cos
  Trigonometric Function3 : Trigonometry  Operator=cos
  Trigonometric Function4 : Trigonometry
  Trigonometric Function5 : Trigonometry
  q : Outport
  d : Outport  Port=2
  0 : Outport  Port=3
  wires:
  Product1/1 -> Sum4/2
  c/1 -> Product9/1, Product6/1, Product2/1
  Constant1/1 -> Product9/2, Product8/2, Product7/2
  Sum2/1 -> Trigonometric Function4/1, Trigonometric Function2/1
  Constant2/1 -> Product11/2, Product10/2, Product3/2
  b/1 -> Product8/1, Product5/1, Product1/1
  Product11/1 -> 0/1
  theta_r/1 -> Sum3/2, Sum2/1, Trigonometric Function1/1, Trigonometric Function/1
  Trigonometric Function2/1 -> Product1/2
  Trigonometric Function5/1 -> Product6/2
  Product6/1 -> Sum5/3
  Trigonometric Function1/1 -> Product4/2
  Constant/1 -> Sum3/1, Sum2/2
  Sum5/1 -> Product10/1
  Product3/1 -> q/1
  Sum4/1 -> Product3/1
  Trigonometric Function3/1 -> Product2/2
  Trigonometric Function/1 -> Product/2
  a/1 -> Product7/1, Product4/1, Product/1
  Product10/1 -> d/1
  Trigonometric Function4/1 -> Product5/2
  Product/1 -> Sum4/1
  Product7/1 -> Sum6/1
  Sum3/1 -> Trigonometric Function5/1, Trigonometric Function3/1
  Product2/1 -> Sum4/3
  Product9/1 -> Sum6/3
  Product5/1 -> Sum5/2
  Product4/1 -> Sum5/1
  Sum6/1 -> Product11/1
  Product8/1 -> Sum6/2

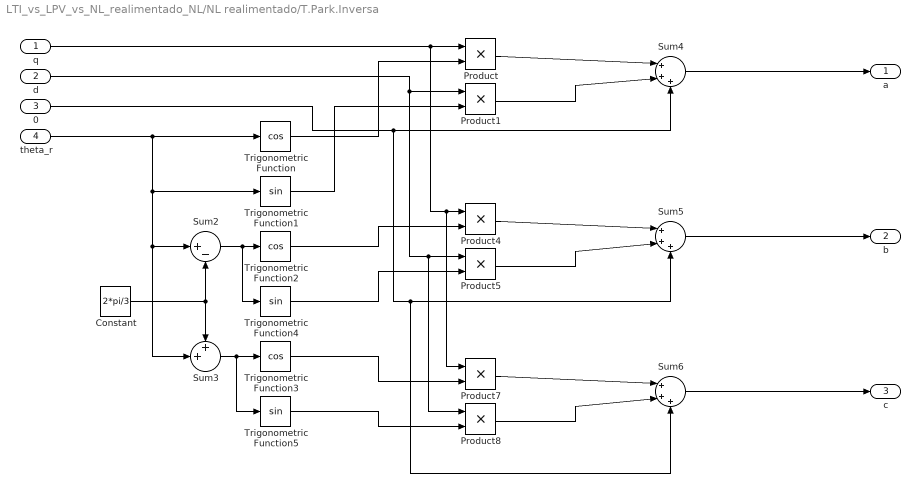
== system LTI_vs_LPV_vs_NL_realimentado_NL/NL realimentado/T.Park.Inversa ==
  q : Inport
  d : Inport  Port=2
  0 : Inport  Port=3
  theta_r : Inport  Port=4
  Constant : Constant  Value=2*pi/3
  Product{,1,4..5,7..8} (6 alike) : Product
  Sum2 : Sum  Inputs=|+-
  Sum3 : Sum  Inputs=++|
  Sum4 : Sum  Inputs=|+++
  Sum5 : Sum  Inputs=|+++
  Sum6 : Sum  Inputs=|+++
  Trigonometric Function : Trigonometry  Operator=cos
  Trigonometric Function1 : Trigonometry
  Trigonometric Function2 : Trigonometry  Operator=cos
  Trigonometric Function3 : Trigonometry  Operator=cos
  Trigonometric Function4 : Trigonometry
  Trigonometric Function5 : Trigonometry
  a : Outport
  b : Outport  Port=2
  c : Outport  Port=3
  wires:
  Constant/1 -> Sum3/1, Sum2/2
  theta_r/1 -> Sum3/2, Sum2/1, Trigonometric Function1/1, Trigonometric Function/1
  Trigonometric Function3/1 -> Product7/2
  d/1 -> Product8/1, Product5/1, Product1/1
  0/1 -> Sum4/3, Sum5/3, Sum6/3
  Product8/1 -> Sum6/2
  Product7/1 -> Sum6/1
  q/1 -> Product7/1, Product4/1, Product/1
  Sum3/1 -> Trigonometric Function5/1, Trigonometric Function3/1
  Trigonometric Function5/1 -> Product8/2
  Sum6/1 -> c/1
  Product1/1 -> Sum4/2
  Sum2/1 -> Trigonometric Function4/1, Trigonometric Function2/1
  Sum4/1 -> a/1
  Sum5/1 -> b/1
  Trigonometric Function1/1 -> Product1/2
  Product5/1 -> Sum5/2
  Trigonometric Function2/1 -> Product4/2
  Product4/1 -> Sum5/1
  Product/1 -> Sum4/1
  Trigonometric Function/1 -> Product/2
  Trigonometric Function4/1 -> Product5/2

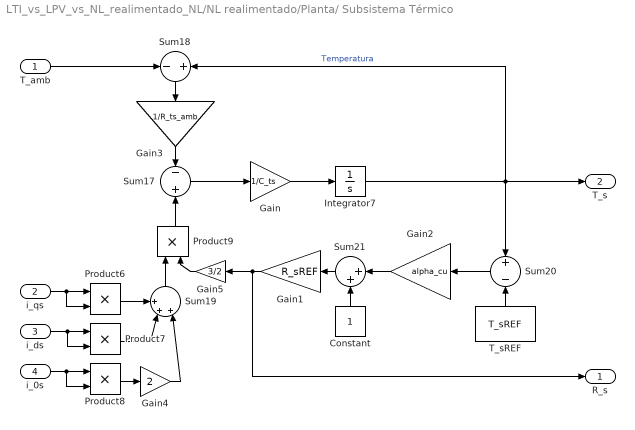
== system LTI_vs_LPV_vs_NL_realimentado_NL/NL realimentado/Planta/	Subsistema Térmico ==
  T_amb : Inport
  i_qs : Inport  Port=2
  i_ds : Inport  Port=3
  i_0s : Inport  Port=4
  Constant : Constant
  Gain : Gain  Gain=1/C_ts
  Gain1 : Gain  Gain=R_sREF
  Gain2 : Gain  Gain=alpha_cu
  Gain3 : Gain  Gain=1/R_ts_amb
  Gain4 : Gain  Gain=2
  Gain5 : Gain  Gain=3/2
  Integrator7 : Integrator  InitialCondition=T_s_o
  Product{6..9} (4 alike) : Product
  Sum17 : Sum  Inputs=-+
  Sum18 : Sum  Inputs=-+
  Sum19 : Sum  Inputs=+++|
  Sum20 : Sum  Inputs=+-
  Sum21 : Sum  Inputs=|++
  T_sREF : Constant  Value=T_sREF
  R_s : Outport
  T_s : Outport  Port=2
  wires:
  Gain4/1 -> Sum19/3
  Integrator7/1 -> Sum18/2, T_s/1, Sum20/1  "Temperatura"
  Sum21/1 -> Gain1/1
  i_ds/1 -> Product7/2, Product7/1
  Product8/1 -> Gain4/1
  Product7/1 -> Sum19/2
  T_amb/1 -> Sum18/1
  Sum18/1 -> Gain3/1
  Product6/1 -> Sum19/1
  Gain/1 -> Integrator7/1
  Product9/1 -> Sum17/2
  Sum17/1 -> Gain/1
  Gain3/1 -> Sum17/1
  T_sREF/1 -> Sum20/2
  Sum20/1 -> Gain2/1
  Gain1/1 -> Gain5/1, R_s/1
  i_qs/1 -> Product6/1, Product6/2
  Sum19/1 -> Product9/1
  Gain2/1 -> Sum21/1
  i_0s/1 -> Product8/2, Product8/1
  Constant/1 -> Sum21/2
  Gain5/1 -> Product9/2

== system LTI_vs_LPV_vs_NL_realimentado_NL/NL realimentado/Planta/Subsistema Mecánico ==
  T_m : Inport
  T_l : Inport  Port=2
  Gain : Gain  Gain=1/r
  Gain3 : Gain  Gain=1/J_eq
  Gain4 : Gain  Gain=b_eq
  Integrator1 : Integrator
  Integrator2 : Integrator
  Sum1 : Sum  Inputs=-+-
  omega_m : Outport
  theta_m : Outport  Port=2
  wires:
  Integrator2/1 -> theta_m/1  "theta_m"
  Gain4/1 -> Sum1/3
  T_m/1 -> Sum1/2
  Integrator1/1 -> Gain4/1, omega_m/1, Integrator2/1  "omega_m"
  Gain/1 -> Sum1/1
  Sum1/1 -> Gain3/1
  Gain3/1 -> Integrator1/1
  T_l/1 -> Gain/1

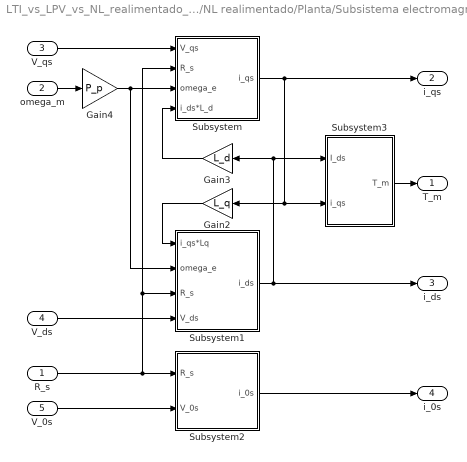
== system LTI_vs_LPV_vs_NL_realimentado_NL/NL realimentado/Planta/Subsistema electromagnético ==
  R_s : Inport
  omega_m : Inport  Port=2
  V_qs : Inport  Port=3
  V_ds : Inport  Port=4
  V_0s : Inport  Port=5
  Gain2 : Gain  Gain=L_q
  Gain3 : Gain  Gain=L_d
  Gain4 : Gain  Gain=P_p
  Subsystem : Subsystem
  Subsystem1 : Subsystem
  Subsystem2 : Subsystem
  Subsystem3 : Subsystem
  T_m : Outport
  i_qs : Outport  Port=2
  i_ds : Outport  Port=3
  i_0s : Outport  Port=4
  wires:
  omega_m/1 -> Gain4/1
  Subsystem/1(i_qs) -> i_qs/1, Subsystem3/2(i_qs), Gain2/1
  Subsystem1/1(i_ds) -> i_ds/1, Subsystem3/1(I_ds), Gain3/1
  Gain2/1 -> Subsystem1/1(i_qs*Lq)
  Gain3/1 -> Subsystem/4(i_ds*L_d)
  Gain4/1 -> Subsystem1/2(omega_e), Subsystem/3(omega_e)
  V_qs/1 -> Subsystem/1(V_qs)
  R_s/1 -> Subsystem/2(R_s), Subsystem1/3(R_s), Subsystem2/1(R_s)
  V_ds/1 -> Subsystem1/4(V_ds)
  V_0s/1 -> Subsystem2/2(V_0s)
  Subsystem2/1(i_0s) -> i_0s/1
  Subsystem3/1(T_m) -> T_m/1

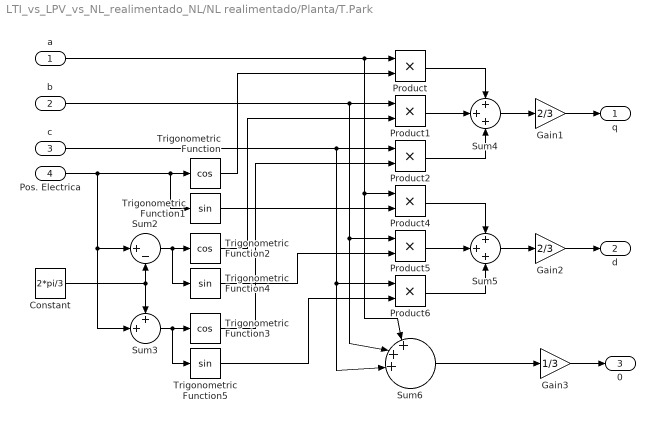
== system LTI_vs_LPV_vs_NL_realimentado_NL/NL realimentado/Planta/T.Park ==
  a : Inport
  b : Inport  Port=2
  c : Inport  Port=3
  Pos. Electrica : Inport  Port=4
  Constant : Constant  Value=2*pi/3
  Gain1 : Gain  Gain=2/3
  Gain2 : Gain  Gain=2/3
  Gain3 : Gain  Gain=1/3
  Product{,1..2,4..6} (6 alike) : Product
  Sum2 : Sum  Inputs=|+-
  Sum3 : Sum  Inputs=++|
  Sum4 : Sum  Inputs=+++
  Sum5 : Sum  Inputs=+++
  Sum6 : Sum  Inputs=|+|+|+||||
  Trigonometric Function : Trigonometry  Operator=cos
  Trigonometric Function1 : Trigonometry
  Trigonometric Function2 : Trigonometry  Operator=cos
  Trigonometric Function3 : Trigonometry  Operator=cos
  Trigonometric Function4 : Trigonometry
  Trigonometric Function5 : Trigonometry
  q : Outport
  d : Outport  Port=2
  0 : Outport  Port=3
  wires:
  Product1/1 -> Sum4/2
  c/1 -> Product2/1, Product6/1, Sum6/3
  Sum2/1 -> Trigonometric Function4/1, Trigonometric Function2/1
  b/1 -> Product1/1, Product5/1, Sum6/2
  Pos. Electrica/1 -> Trigonometric Function/1, Trigonometric Function1/1, Sum3/2, Sum2/1
  Trigonometric Function2/1 -> Product1/2
  Trigonometric Function5/1 -> Product6/2
  Product6/1 -> Sum5/3
  Trigonometric Function1/1 -> Product4/2
  Constant/1 -> Sum3/1, Sum2/2
  Sum5/1 -> Gain2/1
  Gain1/1 -> q/1
  Sum4/1 -> Gain1/1
  Trigonometric Function3/1 -> Product2/2
  Trigonometric Function/1 -> Product/2
  a/1 -> Product4/1, Sum6/1, Product/1
  Trigonometric Function4/1 -> Product5/2
  Product/1 -> Sum4/1
  Sum3/1 -> Trigonometric Function5/1, Trigonometric Function3/1
  Product2/1 -> Sum4/3
  Product5/1 -> Sum5/2
  Product4/1 -> Sum5/1
  Sum6/1 -> Gain3/1
  Gain3/1 -> 0/1
  Gain2/1 -> d/1

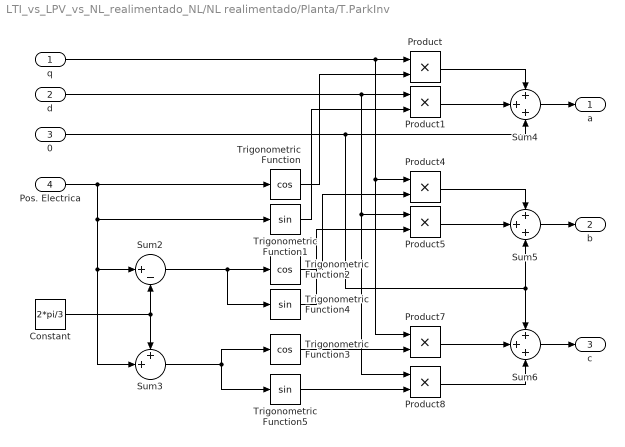
== system LTI_vs_LPV_vs_NL_realimentado_NL/NL realimentado/Planta/T.ParkInv ==
  q : Inport
  d : Inport  Port=2
  0 : Inport  Port=3
  Pos. Electrica : Inport  Port=4
  Constant : Constant  Value=2*pi/3
  Product{,1,4..5,7..8} (6 alike) : Product
  Sum2 : Sum  Inputs=|+-
  Sum3 : Sum  Inputs=++|
  Sum4 : Sum  Inputs=+++
  Sum5 : Sum  Inputs=+++
  Sum6 : Sum  Inputs=+++
  Trigonometric Function : Trigonometry  Operator=cos
  Trigonometric Function1 : Trigonometry
  Trigonometric Function2 : Trigonometry  Operator=cos
  Trigonometric Function3 : Trigonometry  Operator=cos
  Trigonometric Function4 : Trigonometry
  Trigonometric Function5 : Trigonometry
  a : Outport
  b : Outport  Port=2
  c : Outport  Port=3
  wires:
  Constant/1 -> Sum3/1, Sum2/2
  Pos. Electrica/1 -> Sum3/2, Sum2/1, Trigonometric Function1/1, Trigonometric Function/1
  Trigonometric Function3/1 -> Product7/2
  d/1 -> Product8/1, Product5/1, Product1/1
  0/1 -> Sum6/1, Sum5/3, Sum4/3
  Product8/1 -> Sum6/3
  Product7/1 -> Sum6/2
  q/1 -> Product7/1, Product4/1, Product/1
  Sum3/1 -> Trigonometric Function5/1, Trigonometric Function3/1
  Trigonometric Function5/1 -> Product8/2
  Sum6/1 -> c/1
  Product1/1 -> Sum4/2
  Sum2/1 -> Trigonometric Function4/1, Trigonometric Function2/1
  Sum4/1 -> a/1
  Sum5/1 -> b/1
  Trigonometric Function1/1 -> Product1/2
  Product5/1 -> Sum5/2
  Trigonometric Function2/1 -> Product4/2
  Product4/1 -> Sum5/1
  Product/1 -> Sum4/1
  Trigonometric Function/1 -> Product/2
  Trigonometric Function4/1 -> Product5/2

== system LTI_vs_LPV_vs_NL_realimentado_NL/NL realimentado/Planta/Subsistema electromagnético/Subsystem ==
  V_qs : Inport
  R_s : Inport  Port=2
  omega_e : Inport  Port=3
  i_ds*L_d : Inport  Port=4
  Constant : Constant  Value=lambda_m
  Gain8 : Gain  Gain=1/L_q
  Integrator3 : Integrator
  Product : Product
  Product5 : Product
  Sum3 : Sum  Inputs=||+--
  Sum4 : Sum  Inputs=|++
  i_qs : Outport
  wires:
  Constant/1 -> Sum4/2
  Product5/1 -> Sum3/3
  V_qs/1 -> Sum3/1
  i_ds*L_d/1 -> Sum4/1
  Product/1 -> Sum3/2
  Gain8/1 -> Integrator3/1
  Integrator3/1 -> Product5/1, i_qs/1  "i_qs"
  Sum4/1 -> Product/2
  Sum3/1 -> Gain8/1
  R_s/1 -> Product5/2
  omega_e/1 -> Product/1

== system LTI_vs_LPV_vs_NL_realimentado_NL/NL realimentado/Planta/Subsistema electromagnético/Subsystem1 ==
  i_qs*Lq : Inport
  omega_e : Inport  Port=2
  R_s : Inport  Port=3
  V_ds : Inport  Port=4
  Gain : Gain  Gain=1/L_d
  Integrator4 : Integrator
  Product10 : Product
  Product2 : Product
  Sum5 : Sum  Inputs=||++-
  i_ds : Outport
  wires:
  Product10/1 -> Sum5/3
  i_qs*Lq/1 -> Product2/1
  Gain/1 -> Integrator4/1
  V_ds/1 -> Sum5/1
  Sum5/1 -> Gain/1
  R_s/1 -> Product10/2
  Product2/1 -> Sum5/2
  omega_e/1 -> Product2/2
  Integrator4/1 -> i_ds/1, Product10/1  "i_ds"

== system LTI_vs_LPV_vs_NL_realimentado_NL/NL realimentado/Planta/Subsistema electromagnético/Subsystem2 ==
  R_s : Inport
  V_0s : Inport  Port=2
  Gain1 : Gain  Gain=1/L_ls
  Integrator5 : Integrator
  Product11 : Product
  Sum6 : Sum  Inputs=|+-
  i_0s : Outport
  wires:
  Integrator5/1 -> i_0s/1, Product11/1  "i_0s"
  Product11/1 -> Sum6/2
  R_s/1 -> Product11/2
  Sum6/1 -> Gain1/1
  Gain1/1 -> Integrator5/1
  V_0s/1 -> Sum6/1

== system LTI_vs_LPV_vs_NL_realimentado_NL/NL realimentado/Planta/Subsistema electromagnético/Subsystem3 ==
  I_ds : Inport
  i_qs : Inport  Port=2
  Gain5 : Gain  Gain=L_d-L_q
  Gain6 : Gain  Gain=3*P_p/2
  Gain7 : Gain  Gain=lambda_m
  Product1 : Product
  Sum2 : Sum  Inputs=|++
  T_m : Outport
  wires:
  Sum2/1 -> Gain6/1
  Gain7/1 -> Sum2/1
  I_ds/1 -> Product1/2
  Gain5/1 -> Sum2/2
  i_qs/1 -> Product1/1, Gain7/1
  Gain6/1 -> T_m/1
  Product1/1 -> Gain5/1
